simulink model "PMSM_FOC_Tractio"  (R2019b)
settings: Solver=FixedStepAuto  StartTime=0.0  StopTime=10  RelTol=1e-3
model workspace (MAT data in the model file):
  wc : Simulink.Parameter (value not decoded)
values from neighbouring files (symbols this model uses):
  CL_Param = tmp_CL_Param    [PMSM_Parameters.m]
  Cosine_table = [1,0.999995293095708,0.999990587122738,0.999985881149769,0.999981174245477,0.999967055395246,0.999952936545014,0.999938818626106,0.999924698844552,0.999901168979704,0.999877639114857,0.999854108318687,0.999830577522516,0.999797635711730,0.999764694832265,0.999731753021479,0.999698810279369,0.999656459316611,0.999614108353853,0.999571758322418,0.999529405497015,0.999477646313608,0.999425887130201,0 ...(+75635 chars)    [Motor_Table.m]
  ctrlParamsPI = tmp_ctrlParamsPI    [PMSM_Parameters.m]
  Flux_weak = tmp_Fluxweak_struct    [PMSM_Parameters.m]
  Hall_Parameter = tmp_Hall_struct    [PMSM_Parameters.m]
  HFI = tmp_HFI_struct    [PMSM_Parameters.m]
  inverter = struct    [PMSM_Parameters.m]
  MTPA_id_table = [-1.39452500000000,-1.36697494250000,-1.33970177000000,-1.31270548250000,-1.28598608000000,-1.25954356250000,-1.23337793000000,-1.20748918250000,-1.18187732000000,-1.15654234250000,-1.13148425000000,-1.10670304250000,-1.08219872000000,-1.05797128250000,-1.03402073000000,-1.01034706250000,-0.986950280000000,-0.963830382500000,-0.940987370000000,-0.918421242500000,-0.896132000000000,-0.8741196425000 ...(+3439 chars)    [Motor_Table.m]
  MTPA_iq_table = [-10.2740250000000,-10.1791705677750,-10.0840783722000,-9.98875081492500,-9.89319029760000,-9.79739922187500,-9.70137998940000,-9.60513500182500,-9.50866666080000,-9.41197736797500,-9.31506952500000,-9.21794553352500,-9.12060779520000,-9.02305871167500,-8.92530068460000,-8.82733611562500,-8.72916740640000,-8.63079695857500,-8.53222717380000,-8.43346045372500,-8.33449920000000,-8.23534581427500,-8. ...(+3121 chars)    [Motor_Table.m]
  MTPA_Te_Max = single(1.50)    [Motor_Table.m]
  MTPA_Te_Min = single(-1.50)    [Motor_Table.m]
  OPL_Param = tmp_OPL_Param    [PMSM_Parameters.m]
  pmsm = struct    [PMSM_Parameters.m]
  Resolver_Parameter = tmp_Resolver_struct    [PMSM_Parameters.m]
  Sine_table = [0,0.00153398793190718,0.00306797679513693,0.00460196565836668,0.00613595545291901,0.00766988657414913,0.00920381769537926,0.0107377488166094,0.0122716808691621,0.0138054965063930,0.0153393121436238,0.0168731296434999,0.0184069443494082,0.0199405867606401,0.0214742291718721,0.0230078706517816,0.0245415139943361,0.0260749254375696,0.0276083368808031,0.0291417483240366,0.0306751597672701,0.032208281 ...(+75648 chars)    [Motor_Table.m]
  SMO = temp_SMO    [PMSM_Parameters.m]
undefined symbols (not defined in the file or in its folder): DiscIntNeverNeededParam, Kiv, Kiw, Kpv, Kpw, magnitude, sigbuilder_block, SVPWM, Vdc
libraries: powerlib x29, fl_lib x18, simulink x10, nesl_utility x7, eeGeneralControl x4, dspstat3 x3, eeDiscretePi x2, powerlib_extras x1, ee_lib x1
(part 5 of 6)

== system PMSM_FOC_Tractio/Motor_Control/Motor_Control_Funtion/FOC_Control_100us/FOC/Angle_set/Subsystem/Subsystem1 ==
  HFI_Angle : Inport
  Action Port : ActionPort  ActionPortLabel=if(u1 ==3)
  Out1 : Outport
  wires:
  HFI_Angle/1 -> Out1/1

== system PMSM_FOC_Tractio/Motor_Control/Motor_Control_Funtion/FOC_Control_100us/FOC/Angle_set/Subsystem/Subsystem2 ==
  IPD_Angle : Inport
  Action Port : ActionPort  ActionPortLabel=elseif(u1 <3)
  Out1 : Outport
  wires:
  IPD_Angle/1 -> Out1/1

== system PMSM_FOC_Tractio/Motor_Control/Motor_Control_Funtion/FOC_Control_100us/FOC/Flux_weakening /Subsystem/Flux_weak ==
  note: sqrt(Ud*Ud+Uq*Uq)<=Udc/sqrt(3)
  Vd : Inport
  Vq : Inport  Port=2
  id_input : Inport  Port=3
  Iq_input : Inport  Port=4
  Add1 : Sum  OutDataTypeStr=Inherit: Same as first input
  Constant : Constant  Value=pmsm.RatedVoltage/sqrt(3)  OutDataTypeStr=single  SampleTime=-1
  Fcn : Fcn  Expr=sqrt(u(1)^2+u(2)^2)
  ID_Control : Subsystem
  Mux : Mux  Inputs=2
  Sum1 : Sum  Inputs=|-+
  Id_ref : Outport
  iq_ref : Outport  Port=2
  wires:
  Constant/1 -> Sum1/2
  Sum1/1 -> ID_Control/1(Err)
  Mux/1 -> Fcn/1
  Fcn/1 -> Sum1/1
  Vq/1 -> Mux/2
  Iq_input/1 -> iq_ref/1
  id_input/1 -> Add1/1
  Vd/1 -> Mux/1
  Add1/1 -> Id_ref/1
  ID_Control/1(PI_Out) -> Add1/2

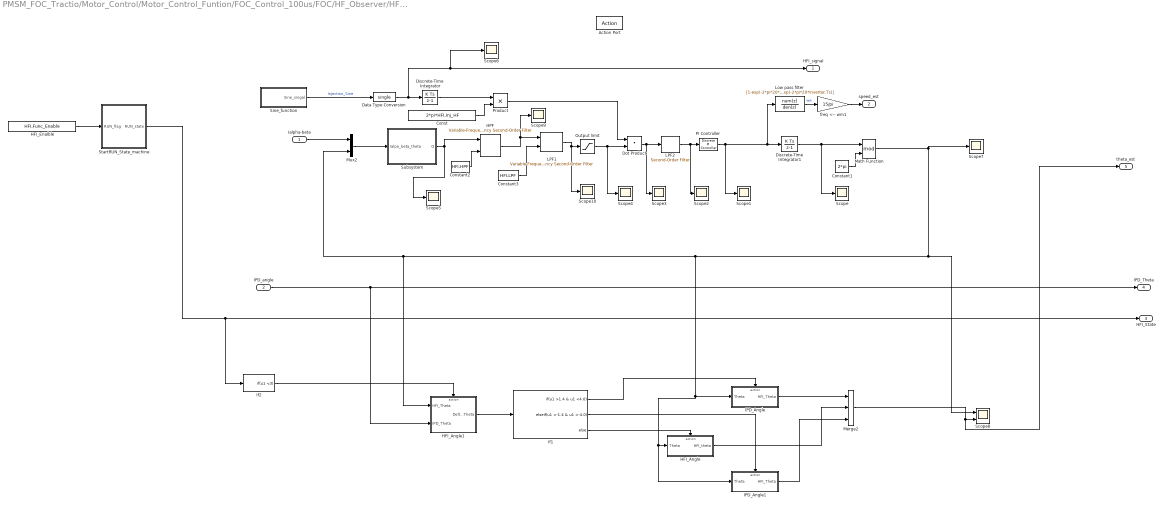
== system PMSM_FOC_Tractio/Motor_Control/Motor_Control_Funtion/FOC_Control_100us/FOC/HF_Observer/HFI_Function/HFI ==
  Ialpha-beta : Inport
  IPD_angle : Inport  Port=2
  Action Port : ActionPort  ActionPortLabel=case [ 3 ]:
  Const : Constant  Value=2*pi*HFI.Inj_HF  OutDataTypeStr=single
  Constant1 : Constant  Value=2*pi  OutDataTypeStr=single
  Constant2 : Constant  Value=HFI.HPF  OutDataTypeStr=single
  Constant3 : Constant  Value=HFI.LPF  OutDataTypeStr=single
  Data Type Conversion : DataTypeConversion  OutDataTypeStr=single
  Discrete-Time Integrator : DiscreteIntegrator  SampleTime=-1  ICPrevOutput=DiscIntNeverNeededParam  ICPrevScaledInput=DiscIntNeverNeededParam
  Discrete-Time Integrator1 : DiscreteIntegrator  SampleTime=-1  ICPrevOutput=DiscIntNeverNeededParam  ICPrevScaledInput=DiscIntNeverNeededParam
  Dot Product : DotProduct  InputSameDT=on  OutDataTypeStr=Inherit: Inherit via internal rule
  HFI_Angle : Subsystem
  HFI_Angle1 : Subsystem
  HFI_Enalble : Constant  Value=HFI.Func_Enable  OutDataTypeStr=uint8
  HPF : eeGeneralControl/Variable-Frequency Second-Order Filter  FilterType=High-pass  fn=HFI.HPF  Zeta=single(0.707)  Ts=-1  A0=0  Ph0=0  f0=0  b0=0
      settings: SourceProductName=Simscape Electrical  SourceProductBaseCode=PS
  IPD_Angle : Subsystem
  IPD_Angle1 : Subsystem
  If1 : If  IfExpression=u1 >1.4 & u1 <4.0  ElseIfExpressions=u1 <-1.4 & u1 >-4.0
  If2 : If  IfExpression=u1 <3  ShowElse=off
  LPF1 : eeGeneralControl/Variable-Frequency Second-Order Filter  FilterType=Low-pass  fn=HFI.LPF  Zeta=single(0.707)  Ts=-1  A0=0  Ph0=0  f0=0  b0=0
      settings: SourceProductName=Simscape Electrical  SourceProductBaseCode=PS
  LPF2 : eeGeneralControl/Second-Order Filter  FilterType=Low-pass  fn=100  Zeta=single(0.707)  Ts=-1  A0=0  Ph0=0  f0=0  b0=0
      settings: SourceProductName=Simscape Electrical  SourceProductBaseCode=PS
  Low pass filter : DiscreteTransferFcn  Numerator=[1-exp(-2*pi*20*inverter.Ts)]  Denominator=[1 -exp(-2*pi*20*inverter.Ts)]
  Math Function : Math  Operator=mod  SaturateOnIntegerOverflow=on
  Merge2 : Merge  Inputs=3
  Mux2 : Mux  Inputs=2
  Output limit : Saturate
  PI Controller : powerlib_extras/Discrete  Control Blocks/Discrete PI Controller  Kp=HFI.PI_Kp  Ki=HFI.PI_Ki  Par_Limits=[100*2*pi -100*2*pi]  Init=0  Ts=-1
      settings: SourceProductName=Simscape Electrical
  Product : Product
  Scope{,1..7,9..10} (10 alike) : Scope
  Scope8 : Scope  NumInputPorts=2
  Sine_function : Subsystem
      settings: RTWSystemCode=Nonreusable function  RTWFcnNameOpts=Use subsystem name
  StartRUN_State_machine : Stateflow chart  BlockKeywords=__PRM__SERIALIZED__DATA__:Stateflow Chart,Stateflow Diagram  TreatAsAtomicUnit=on
      settings: RTWSystemCode=Nonreusable function  RTWFcnNameOpts=Use subsystem name
  Subsystem : Subsystem
  freq <-- wm1 : Gain  Gain=15/pi
  HFI_signal : Outport
  speed_est : Outport  Port=2
  HFI_State : Outport  Port=3
  IPD_Theta : Outport  Port=4
  theta_est : Outport  Port=5
  wires:
  Mux2/1 -> Subsystem/1(Ialpa_beta_theta)
  Ialpha-beta/1 -> Mux2/1
  Subsystem/1(Q) -> HPF/1, Scope5/1
  freq <-- wm1/1 -> speed_est/1
  Discrete-Time Integrator1/1 -> Scope/1, Math Function/1
  LPF1/1 -> Scope10/1, Output limit/1
  LPF2/1 -> Scope2/1, PI Controller/1
  Low pass filter/1 -> freq <-- wm1/1  "we"
  HPF/1 -> LPF1/1, Scope9/1
  Discrete-Time Integrator/1 -> Product/1
  Product/1 -> Dot Product/1
  Dot Product/1 -> LPF2/1, Scope3/1
  Constant1/1 -> Math Function/2
  Output limit/1 -> Scope4/1, Dot Product/2
  Const/1 -> Product/2
  Sine_function/1(Sine_singal) -> Data Type Conversion/1  "Injection_Sine"
  Data Type Conversion/1 -> Scope6/1, HFI_signal/1, Discrete-Time Integrator/1
  HFI_Enalble/1 -> StartRUN_State_machine/1(RUN_flag)
  StartRUN_State_machine/1(RUN_state) -> If2/1, HFI_State/1
  IPD_angle/1 -> HFI_Angle1/2(IPD_Theta), IPD_Theta/1
  Math Function/1 -> IPD_Angle1/1(Theta), HFI_Angle/1(Theta), IPD_Angle/1(Theta), HFI_Angle1/1(HFI_Theta), Mux2/2, Scope8/1, Scope7/1
  PI Controller/1 -> Low pass filter/1, Discrete-Time Integrator1/1, Scope1/1
  If1/1 -> IPD_Angle/Action
  HFI_Angle/1(HFI_theta) -> Merge2/2
  If1/3 -> HFI_Angle/Action
  IPD_Angle/1(HFI_Theta) -> Merge2/1
  HFI_Angle1/1(Delta_Theta) -> If1/1
  If2/1 -> HFI_Angle1/Action
  Merge2/1 -> theta_est/1, Scope8/2
  If1/2 -> IPD_Angle1/Action
  IPD_Angle1/1(HFI_Theta) -> Merge2/3
  Constant2/1 -> HPF/2
  Constant3/1 -> LPF1/2

== system PMSM_FOC_Tractio/Motor_Control/Motor_Control_Funtion/FOC_Control_100us/FOC/HF_Observer/HFI_Function/IPD ==
  Iabc : Inport  PortDimensions=3
  Action Port : ActionPort  ActionPortLabel=case [ 1 ]:
  7 : Fcn  Expr=u[1]*u[3]
  8 : Fcn  Expr=u[1]*u[2]
  Constant : Constant  Value=HFI.IPD_V
  Demux1 : Demux  Outputs=3
  HF_Angle : Subsystem
  Mux : Mux  Inputs=3
  Scope : Scope
  Sine_Cosine : Subsystem  TreatAsAtomicUnit=on
      settings: RTWSystemCode=Nonreusable function  RTWFcnNameOpts=Use subsystem name
  Theta_cacl : Subsystem
      settings: RTWSystemCode=Nonreusable function
  Ualpha : Outport
  Ubeta : Outport  Port=2
  Theta : Outport  Port=3
  wires:
  Sine_Cosine/1(Sin) -> Mux/2
  Sine_Cosine/2(Cos) -> Mux/3
  Constant/1 -> Mux/1
  Mux/1 -> 8/1, 7/1
  7/1 -> Ualpha/1
  8/1 -> Ubeta/1
  Iabc/1 -> Scope/1, Demux1/1  "Phase_CurrentABC"
  HF_Angle/1(Theta_V) -> Sine_Cosine/1(P)
  Demux1/3 -> Theta_cacl/3(Ic)
  Demux1/2 -> Theta_cacl/2(Ib)
  Theta_cacl/1(Theta) -> Theta/1
  Demux1/1 -> Theta_cacl/1(Ia)

== system PMSM_FOC_Tractio/Motor_Control/Motor_Control_Funtion/FOC_Control_100us/FOC/HF_Observer/HFI_Function/NS ==
  Id : Inport
  Theta : Inport  Port=2
  Action Port : ActionPort  ActionPortLabel=case [ 2 ]:
  Abs : Abs
  Abs1 : Abs
  Data Type Conversion : DataTypeConversion
  Delay : Delay  DelayLength=1  InitialCondition=0
  Delay1 : Delay  DelayLength=1  InitialCondition=0
  HFI_Enalble : Constant  Value=HFI.Func_Enable  OutDataTypeStr=uint8
  Merge : Merge  Inputs=5
  Merge1 : Merge  Inputs=5
  NS_State_machine : Stateflow chart  BlockKeywords=__PRM__SERIALIZED__DATA__:Stateflow Chart,Stateflow Diagram  TreatAsAtomicUnit=on
      settings: RTWSystemCode=Nonreusable function  RTWFcnNameOpts=Use subsystem name
  Scope1 : Scope  NumInputPorts=2
  Switch Case1 : SwitchCase  CaseConditions={1,2,3,4,5}  ShowDefaultCase=off
  Ud_inject_1 : Subsystem
  Ud_inject_2 : Subsystem
  Ud_inject_3 : Subsystem
  Ud_inject_4 : Subsystem
  Ud_inject_5 : Subsystem
  Ualpha : Outport
  Ubeta : Outport  Port=2
  IPD_Angle : Outport  Port=3
  Angle_RUN : Outport  Port=4
  wires:
  HFI_Enalble/1 -> NS_State_machine/1(NS_flag1)
  NS_State_machine/1(NS_state) -> Switch Case1/1
  Id/1 -> Ud_inject_2/1(Id), Ud_inject_4/1(Id)
  Merge/1 -> Scope1/1, Ualpha/1
  Ud_inject_2/1(Ualpha) -> Merge/1
  Ud_inject_4/1(Ualpha) -> Merge/2
  Merge1/1 -> Scope1/2, Ubeta/1
  Ud_inject_2/2(Ubeta) -> Merge1/1
  Ud_inject_4/2(Ubeta) -> Merge1/2
  Ud_inject_4/3(Id_out) -> Delay1/1
  Ud_inject_2/3(Id_out) -> Delay/1
  Ud_inject_1/1(Ualpha) -> Merge/3
  Ud_inject_1/2(Ubeta) -> Merge1/3
  Ud_inject_3/1(Ualpha) -> Merge/4
  Ud_inject_3/2(Ubeta) -> Merge1/4
  Switch Case1/1 -> Ud_inject_1/Action
  Switch Case1/2 -> Ud_inject_2/Action
  Theta/1 -> Ud_inject_4/2(Theta), Ud_inject_2/2(Theta), Ud_inject_1/1(Theta), Ud_inject_5/1(Theta), Ud_inject_3/1(Theta)
  Switch Case1/3 -> Ud_inject_3/Action
  Switch Case1/4 -> Ud_inject_4/Action
  Switch Case1/5 -> Ud_inject_5/Action
  Ud_inject_5/1(Ualpha) -> Merge/5
  Ud_inject_5/2(Ubeta) -> Merge1/5
  Abs/1 -> Ud_inject_5/2(Id1)
  Abs1/1 -> Ud_inject_5/3(Id2)
  Ud_inject_5/3(IPD_Angle) -> Data Type Conversion/1, IPD_Angle/1
  Delay/1 -> Abs/1
  Delay1/1 -> Abs1/1
  Data Type Conversion/1 -> Angle_RUN/1

== system PMSM_FOC_Tractio/Motor_Control/Motor_Control_Funtion/Angle_Speed_100us/SpeedAndAngle/ACC_OMG/BLDC/Control/Commutation ==
  Hall : Inport
  Bias : Bias  Bias=-1
  Bit concatenate : Subsystem
  Data Type Conversion : DataTypeConversion
  Direct Lookup Table (n-D)2 : LookupNDDirect  InputsSelectThisObjectFromTable=Vector  Table=[0 0 0 1 1 0;0 1 1 0 0 0;0 1 0 0 0 1;1 0 0 0 1 0;1 0 1 0 0 0;0 0 0 1 0 1]
  Scope : Scope
  S : Outport  VectorParamsAs1DForOutWhenUnconnected=off
  wires:
  Hall/1 -> Bit concatenate/1(u)
  Bit concatenate/1(y) -> Data Type Conversion/1
  Direct Lookup Table (n-D)2/1 -> S/1
  Data Type Conversion/1 -> Bias/1
  Bias/1 -> Scope/1, Direct Lookup Table (n-D)2/1

== system PMSM_FOC_Tractio/Motor_Control/Motor_Control_Funtion/Angle_Speed_100us/SpeedAndAngle/ACC_OMG/BLDC/Control/Speed_Control ==
  Err : Inport
  Action Port : ActionPort  ActionPortLabel=if(u1==3)
  Add : Sum
  Cons : Constant  Value=0  OutDataTypeStr=single
  Discrete-Time Integrator : DiscreteIntegrator  SampleTime=-1  ICPrevOutput=DiscIntNeverNeededParam  ICPrevScaledInput=DiscIntNeverNeededParam
  Ki : Constant  Value=17.72  OutDataTypeStr=single
  Kp : Constant  Value=0.7476  OutDataTypeStr=single
  Product : Product
  Product1 : Product
  Relational Operator1 : RelationalOperator  Operator===  OutDataTypeStr=boolean  RndMeth=Simplest
  Saturation : Saturate  UpperLimit=4200  LowerLimit=0
  Scope : Scope
  Switch : Switch  Criteria=u2 > Threshold
  Unit Delay3 : UnitDelay  SampleTime=-1  HasFrameUpgradeWarning=on
  PI_Out : Outport
  wires:
  Kp/1 -> Product/1
  Err/1 -> Switch/1, Product/2
  Switch/1 -> Product1/2
  Product1/1 -> Discrete-Time Integrator/1
  Product/1 -> Add/1
  Add/1 -> Relational Operator1/1, Saturation/1
  Saturation/1 -> Relational Operator1/2, PI_Out/1
  Discrete-Time Integrator/1 -> Add/2, Scope/1
  Relational Operator1/1 -> Unit Delay3/1
  Ki/1 -> Product1/1
  Unit Delay3/1 -> Switch/2
  Cons/1 -> Switch/3

== system PMSM_FOC_Tractio/Motor_Control/Motor_Control_Funtion/Angle_Speed_100us/SpeedAndAngle/Subsystem/Subsystem1/Commutation/Bit concatenate ==
  u : Inport
  Gain : Gain  Gain=[4 2 1]  Multiplication=Matrix(K*u)
  Sum of Elements : Sum  Inputs=+
  y : Outport  VectorParamsAs1DForOutWhenUnconnected=off
  wires:
  u/1 -> Gain/1
  Gain/1 -> Sum of Elements/1
  Sum of Elements/1 -> y/1

== system PMSM_FOC_Tractio/Motor_Control/Motor_Control_Funtion/FOC_Control_100us/FOC/Flux_weakening /Subsystem/Flux_weak/ID_Control ==
  Err : Inport
  Add : Sum
  Cons : Constant  Value=0  OutDataTypeStr=single
  Discrete-Time Integrator : DiscreteIntegrator  SampleTime=-1  ICPrevOutput=DiscIntNeverNeededParam  ICPrevScaledInput=DiscIntNeverNeededParam
  Ki : Constant  Value=ki  OutDataTypeStr=single
  Kp : Constant  Value=kp  OutDataTypeStr=single
  Product : Product
  Product1 : Product
  Relational Operator1 : RelationalOperator  Operator===  OutDataTypeStr=boolean  RndMeth=Simplest
  Saturation : Saturate  UpperLimit=Id_max  LowerLimit=Id_min
  Switch : Switch  Criteria=u2 > Threshold
  Unit Delay3 : UnitDelay  SampleTime=-1  HasFrameUpgradeWarning=on
  PI_Out : Outport
  wires:
  Kp/1 -> Product/1
  Err/1 -> Switch/1, Product/2
  Switch/1 -> Product1/2
  Product1/1 -> Discrete-Time Integrator/1
  Product/1 -> Add/1
  Add/1 -> Relational Operator1/1, Saturation/1
  Saturation/1 -> Relational Operator1/2, PI_Out/1
  Cons/1 -> Switch/3
  Discrete-Time Integrator/1 -> Add/2
  Relational Operator1/1 -> Unit Delay3/1
  Ki/1 -> Product1/1
  Unit Delay3/1 -> Switch/2

== system PMSM_FOC_Tractio/Motor_Control/Motor_Control_Funtion/FOC_Control_100us/FOC/HF_Observer/HFI_Function/HFI/HFI_Angle ==
  Theta : Inport
  Action Port : ActionPort  ActionPortLabel=else
  HFI_theta : Outport
  wires:
  Theta/1 -> HFI_theta/1

== system PMSM_FOC_Tractio/Motor_Control/Motor_Control_Funtion/FOC_Control_100us/FOC/HF_Observer/HFI_Function/HFI/HFI_Angle1 ==
  HFI_Theta : Inport
  IPD_Theta : Inport  Port=2
  Action Port : ActionPort  ActionPortLabel=if(u1 <3)
  Subtract : Sum  Inputs=+-
  Delta_Theta : Outport
  wires:
  HFI_Theta/1 -> Subtract/1
  IPD_Theta/1 -> Subtract/2
  Subtract/1 -> Delta_Theta/1

== system PMSM_FOC_Tractio/Motor_Control/Motor_Control_Funtion/FOC_Control_100us/FOC/HF_Observer/HFI_Function/HFI/IPD_Angle ==
  Theta : Inport
  Action Port : ActionPort  ActionPortLabel=if(u1 >1.4 & u1 <4.0)
  Angle_calibration : Subsystem  TreatAsAtomicUnit=on
      settings: RTWSystemCode=Nonreusable function  RTWFcnNameOpts=Use subsystem name
  HFI_Theta : Outport
  wires:
  Theta/1 -> Angle_calibration/1(Angle_input)
  Angle_calibration/1(Angle_output) -> HFI_Theta/1

== system PMSM_FOC_Tractio/Motor_Control/Motor_Control_Funtion/FOC_Control_100us/FOC/HF_Observer/HFI_Function/HFI/IPD_Angle1 ==
  Theta : Inport
  Action Port : ActionPort  ActionPortLabel=elseif(u1 <-1.4 & u1 >-4.0)
  Angle_calibration : Subsystem  TreatAsAtomicUnit=on
      settings: RTWSystemCode=Nonreusable function  RTWFcnNameOpts=Use subsystem name
  HFI_Theta : Outport
  wires:
  Theta/1 -> Angle_calibration/1(Angle_input)
  Angle_calibration/1(Angle_output) -> HFI_Theta/1

== system PMSM_FOC_Tractio/Motor_Control/Motor_Control_Funtion/FOC_Control_100us/FOC/HF_Observer/HFI_Function/HFI/Sine_function ==
  A : Gain  Gain=HFI.Inj_HV
  Add : Sum
  Const1 : Constant  Value=2*pi*inverter.Ts*HFI.Inj_HF  OutDataTypeStr=single
  Const2 : Constant  Value=2*pi  OutDataTypeStr=single
  Const3 : Constant  Value=0  OutDataTypeStr=single
  Const4 : Constant  OutDataTypeStr=single
  Delay : Delay  DelayLength=1  InitialCondition=0
  Memory : Memory  InheritSampleTime=on
  Product1 : Product
  Relational Operator1 : RelationalOperator  Operator=<  OutDataTypeStr=boolean  RndMeth=Simplest
  Sine : Lookup_n-D  NumberOfTableDimensions=1  LookupTableObject=''  BreakpointsForDimension1=[0:2*pi/4095:2*pi]  BreakpointsForDimension1FirstPoint=10  BreakpointsForDimension2FirstPoint=10  BreakpointsForDimension1Spacing=12  BreakpointsForDimension2Spacing=12  IndexSearchMethod=Evenly spaced points  Table=Sine_table  InterpMethod=Flat  DiagnosticForOutOfRangeInput=Error  InternalRulePriority=Speed  RndMeth=Simplest  InputSameDT=on
  Switch : Switch  Criteria=u2 > Threshold
  Sine_singal : Outport
  wires:
  Switch/1 -> Product1/1
  Const3/1 -> Switch/3
  Relational Operator1/1 -> Switch/2
  Delay/1 -> Relational Operator1/1
  Const2/1 -> Relational Operator1/2
  Add/1 -> Memory/1, Delay/1
  Sine/1 -> A/1
  Product1/1 -> Sine/1, Add/2
  Memory/1 -> Product1/2
  Const1/1 -> Add/1
  Const4/1 -> Switch/1
  A/1 -> Sine_singal/1

== system PMSM_FOC_Tractio/Motor_Control/Motor_Control_Funtion/FOC_Control_100us/FOC/HF_Observer/HFI_Function/HFI/Subsystem ==
  Ialpa_beta_theta : Inport
  Add2 : Sum  Inputs=-+  OutDataTypeStr=Inherit: Same as first input
  Demux : Demux  Outputs=2
  Demux1 : Demux  Outputs=2
  Produc3t : Product  RndMeth=Simplest  OutDataTypeStr=Inherit: Same as first input
  Product4 : Product  RndMeth=Simplest  OutDataTypeStr=Inherit: Same as first input
  Sine_Cosine : Subsystem
      settings: RTWSystemCode=Nonreusable function  RTWFcnNameOpts=Use subsystem name
  Q : Outport  VectorParamsAs1DForOutWhenUnconnected=off
  wires:
  Add2/1 -> Q/1
  Sine_Cosine/2(Cos) -> Product4/2
  Produc3t/1 -> Add2/1
  Sine_Cosine/1(Sin) -> Produc3t/2
  Product4/1 -> Add2/2
  Demux/1 -> Produc3t/1
  Demux/2 -> Product4/1
  Demux1/1 -> Demux/1
  Demux1/2 -> Sine_Cosine/1(P)
  Ialpa_beta_theta/1 -> Demux1/1

== system PMSM_FOC_Tractio/Motor_Control/Motor_Control_Funtion/FOC_Control_100us/FOC/HF_Observer/HFI_Function/IPD/HF_Angle ==
  Add : Sum
  Const1 : Constant  Value=2*pi*inverter.Ts*HFI.IPD_F  OutDataTypeStr=single
  Const2 : Constant  Value=2*pi  OutDataTypeStr=single
  Const3 : Constant  Value=0  OutDataTypeStr=single
  Const4 : Constant  OutDataTypeStr=single
  Delay : Delay  DelayLength=1  InitialCondition=0
  Memory : Memory  InheritSampleTime=on
  Product1 : Product
  Relational Operator1 : RelationalOperator  Operator=<  OutDataTypeStr=boolean  RndMeth=Simplest
  Switch : Switch  Criteria=u2 > Threshold
  Theta_V : Outport
  wires:
  Switch/1 -> Product1/1
  Delay/1 -> Relational Operator1/1
  Const2/1 -> Relational Operator1/2
  Const3/1 -> Switch/3
  Relational Operator1/1 -> Switch/2
  Const1/1 -> Add/1
  Memory/1 -> Product1/2
  Add/1 -> Memory/1, Delay/1
  Product1/1 -> Theta_V/1, Add/2
  Const4/1 -> Switch/1

== system PMSM_FOC_Tractio/Motor_Control/Motor_Control_Funtion/FOC_Control_100us/FOC/HF_Observer/HFI_Function/IPD/Sine_Cosine ==
  note: Sine Cosine Coefficients
  P : Inport
  Cosine : Lookup_n-D  NumberOfTableDimensions=1  LookupTableObject=''  BreakpointsForDimension1=[0:2*pi/4095:2*pi]  BreakpointsForDimension1FirstPoint=10  BreakpointsForDimension2FirstPoint=10  BreakpointsForDimension1Spacing=12  BreakpointsForDimension2Spacing=12  IndexSearchMethod=Evenly spaced points  Table=Cosine_table  InterpMethod=Flat  DiagnosticForOutOfRangeInput=Error  InternalRulePriority=Speed  RndMeth=Simplest  InputSameDT=on
  Scope : Scope  NumInputPorts=2
  Sine : Lookup_n-D  NumberOfTableDimensions=1  LookupTableObject=''  BreakpointsForDimension1=[0:2*pi/4095:2*pi]  BreakpointsForDimension1FirstPoint=10  BreakpointsForDimension2FirstPoint=10  BreakpointsForDimension1Spacing=12  BreakpointsForDimension2Spacing=12  IndexSearchMethod=Evenly spaced points  Table=Sine_table  InterpMethod=Flat  DiagnosticForOutOfRangeInput=Error  InternalRulePriority=Speed  RndMeth=Simplest  InputSameDT=on
  Sin : Outport  VectorParamsAs1DForOutWhenUnconnected=off
  Cos : Outport  Port=2  VectorParamsAs1DForOutWhenUnconnected=off
  wires:
  P/1 -> Cosine/1, Sine/1  "position"
  Sine/1 -> Scope/1, Sin/1
  Cosine/1 -> Scope/2, Cos/1

== system PMSM_FOC_Tractio/Motor_Control/Motor_Control_Funtion/FOC_Control_100us/FOC/HF_Observer/HFI_Function/IPD/Theta_cacl ==
  Ia : Inport
  Ib : Inport  Port=2
  Ic : Inport  Port=3
  Display{1..3,6} (4 alike) : Display
  Gain1 : Gain  Gain=pi/180
  If Action Subsystem1 : Subsystem  TreatAsAtomicUnit=on
  If Action Subsystem2 : Subsystem  TreatAsAtomicUnit=on
  If Action Subsystem3 : Subsystem  TreatAsAtomicUnit=on
  If Action Subsystem4 : Subsystem  TreatAsAtomicUnit=on
  If Action Subsystem5 : Subsystem  TreatAsAtomicUnit=on
  If Action Subsystem6 : Subsystem  TreatAsAtomicUnit=on
  If1 : If  NumInputs=3  IfExpression=(u1>u3)&(u3>u2)  ElseIfExpressions=(u3>u1)&(u1>u2),(u3>u2)&(u2>u1),(u2>u3)&(u3>u1),(u2>u1)&(u1>u3),(u1>u2)&(u2>u3)  ShowElse=off
  Merge : Merge  Inputs=6
  Mux2 : Mux  Inputs=3
  RMS : dspstat3/RMS  run=on  directionMode=Each column  dimension=1  reset_popup=None
  RMS1 : dspstat3/RMS  run=on  directionMode=Each column  dimension=1  reset_popup=None
  RMS2 : dspstat3/RMS  run=on  directionMode=Each column  dimension=1  InputProcessing=Columns as channels (frame based)  reset_popup=None
  Scope1 : Scope  NumInputPorts=3
  Scope2 : Scope  NumInputPorts=3
  Theta : Outport
  wires:
  Ia/1 -> Scope2/1, RMS/1
  Ib/1 -> Scope2/2, RMS1/1
  Ic/1 -> Scope2/3, RMS2/1
  RMS2/1 -> Mux2/3, If1/3, Display3/1, Scope1/3
  RMS1/1 -> Mux2/2, If1/2, Display2/1, Scope1/2
  RMS/1 -> If1/1, Mux2/1, Display1/1, Scope1/1
  If1/1 -> If Action Subsystem2/Action
  If1/2 -> If Action Subsystem1/Action
  If1/3 -> If Action Subsystem3/Action
  If1/4 -> If Action Subsystem4/Action
  If1/5 -> If Action Subsystem5/Action
  If1/6 -> If Action Subsystem6/Action
  Mux2/1 -> If Action Subsystem6/1(In1), If Action Subsystem5/1(In1), If Action Subsystem4/1(In1), If Action Subsystem3/1(In1), If Action Subsystem1/1(In1), If Action Subsystem2/1(In1)
  If Action Subsystem2/1(Out1) -> Merge/1
  If Action Subsystem1/1(Out1) -> Merge/2
  If Action Subsystem3/1(Out1) -> Merge/3
  If Action Subsystem4/1(Out1) -> Merge/4
  If Action Subsystem5/1(Out1) -> Merge/5
  If Action Subsystem6/1(Out1) -> Merge/6
  Merge/1 -> Gain1/1
  Gain1/1 -> Display6/1, Theta/1

== system PMSM_FOC_Tractio/Motor_Control/Motor_Control_Funtion/FOC_Control_100us/FOC/HF_Observer/HFI_Function/NS/Ud_inject_1 ==
  Theta : Inport
  Action Port : ActionPort  ActionPortLabel=case [ 1 ]:
  1 : Fcn  Expr=u[1]*u[4]-u[2]*u[3]
  2 : Fcn  Expr=u[1]*u[3]+u[2]*u[4]
  Constant : Constant  Value=0  OutDataTypeStr=single
  Constant2 : Constant  Value=0  OutDataTypeStr=single
  Mux : Mux
  Sine_Cosine : Subsystem  TreatAsAtomicUnit=on
      settings: RTWSystemCode=Nonreusable function  RTWFcnNameOpts=Use subsystem name
  Ualpha : Outport
  Ubeta : Outport  Port=2
  wires:
  Constant2/1 -> Mux/2
  Theta/1 -> Sine_Cosine/1(P)
  2/1 -> Ubeta/1
  Sine_Cosine/2(Cos) -> Mux/4
  1/1 -> Ualpha/1
  Constant/1 -> Mux/1
  Mux/1 -> 2/1, 1/1
  Sine_Cosine/1(Sin) -> Mux/3

== system PMSM_FOC_Tractio/Motor_Control/Motor_Control_Funtion/FOC_Control_100us/FOC/HF_Observer/HFI_Function/NS/Ud_inject_2 ==
  Id : Inport
  Theta : Inport  Port=2
  Action Port : ActionPort  ActionPortLabel=case [ 2 ]:
  1 : Fcn  Expr=u[1]*u[4]-u[2]*u[3]
  2 : Fcn  Expr=u[1]*u[3]+u[2]*u[4]
  Constant : Constant  Value=HFI.NS_V  OutDataTypeStr=single
  Constant2 : Constant  Value=0  OutDataTypeStr=single
  Mux : Mux
  Sine_Cosine : Subsystem  TreatAsAtomicUnit=on
      settings: RTWSystemCode=Nonreusable function  RTWFcnNameOpts=Use subsystem name
  Ualpha : Outport
  Ubeta : Outport  Port=2
  Id_out : Outport  Port=3
  wires:
  Constant2/1 -> Mux/2
  Theta/1 -> Sine_Cosine/1(P)
  2/1 -> Ubeta/1
  Sine_Cosine/2(Cos) -> Mux/4
  1/1 -> Ualpha/1
  Constant/1 -> Mux/1
  Mux/1 -> 2/1, 1/1
  Sine_Cosine/1(Sin) -> Mux/3
  Id/1 -> Id_out/1

== system PMSM_FOC_Tractio/Motor_Control/Motor_Control_Funtion/FOC_Control_100us/FOC/HF_Observer/HFI_Function/NS/Ud_inject_3 ==
  Theta : Inport
  Action Port : ActionPort  ActionPortLabel=case [ 3 ]:
  1 : Fcn  Expr=u[1]*u[4]-u[2]*u[3]
  2 : Fcn  Expr=u[1]*u[3]+u[2]*u[4]
  Constant : Constant  Value=0  OutDataTypeStr=single
  Constant2 : Constant  Value=0  OutDataTypeStr=single
  Mux : Mux
  Sine_Cosine : Subsystem  TreatAsAtomicUnit=on
      settings: RTWSystemCode=Nonreusable function  RTWFcnNameOpts=Use subsystem name
  Ualpha : Outport
  Ubeta : Outport  Port=2
  wires:
  Constant2/1 -> Mux/2
  Theta/1 -> Sine_Cosine/1(P)
  2/1 -> Ubeta/1
  Sine_Cosine/2(Cos) -> Mux/4
  1/1 -> Ualpha/1
  Constant/1 -> Mux/1
  Mux/1 -> 2/1, 1/1
  Sine_Cosine/1(Sin) -> Mux/3

== system PMSM_FOC_Tractio/Motor_Control/Motor_Control_Funtion/FOC_Control_100us/FOC/HF_Observer/HFI_Function/NS/Ud_inject_4 ==
  Id : Inport
  Theta : Inport  Port=2
  Action Port : ActionPort  ActionPortLabel=case [ 4 ]:
  1 : Fcn  Expr=u[1]*u[4]-u[2]*u[3]
  2 : Fcn  Expr=u[1]*u[3]+u[2]*u[4]
  Constant : Constant  Value=HFI.NS_V  OutDataTypeStr=single
  Constant2 : Constant  Value=0  OutDataTypeStr=single
  Mux : Mux
  Sine_Cosine : Subsystem  TreatAsAtomicUnit=on
      settings: RTWSystemCode=Nonreusable function
  Theta_limit : Subsystem
      settings: RTWSystemCode=Nonreusable function
  Ualpha : Outport
  Ubeta : Outport  Port=2
  Id_out : Outport  Port=3
  wires:
  Constant2/1 -> Mux/2
  2/1 -> Ubeta/1
  Sine_Cosine/2(Cos) -> Mux/4
  1/1 -> Ualpha/1
  Constant/1 -> Mux/1
  Mux/1 -> 2/1, 1/1
  Sine_Cosine/1(Sin) -> Mux/3
  Id/1 -> Id_out/1
  Theta_limit/1(Angle_output) -> Sine_Cosine/1(P)
  Theta/1 -> Theta_limit/1(Angle_input)

== system PMSM_FOC_Tractio/Motor_Control/Motor_Control_Funtion/FOC_Control_100us/FOC/HF_Observer/HFI_Function/NS/Ud_inject_5 ==
  Theta : Inport
  Id1 : Inport  Port=2
  Id2 : Inport  Port=3
  Action Port : ActionPort  ActionPortLabel=case [ 5 ]:
  1 : Fcn  Expr=u[1]*u[4]-u[2]*u[3]
  2 : Fcn  Expr=u[1]*u[3]+u[2]*u[4]
  Constant : Constant  Value=0  OutDataTypeStr=single
  Constant2 : Constant  Value=0  OutDataTypeStr=single
  If1 : If  NumInputs=2  IfExpression=u1>=u2  ElseIfExpressions=u1<u2  ShowElse=off
  Merge1 : Merge
  Mux : Mux
  Sine_Cosine : Subsystem
      settings: RTWSystemCode=Nonreusable function  RTWFcnNameOpts=Use subsystem name
  Subsystem : Subsystem
  Subsystem1 : Subsystem
  Ualpha : Outport
  Ubeta : Outport  Port=2
  IPD_Angle : Outport  Port=3
  wires:
  Constant2/1 -> Mux/2
  Theta/1 -> Subsystem1/1(In1), Subsystem/1(In1), Sine_Cosine/1(P)
  2/1 -> Ubeta/1
  Sine_Cosine/2(Cos) -> Mux/4
  1/1 -> Ualpha/1
  Constant/1 -> Mux/1
  Mux/1 -> 2/1, 1/1
  Sine_Cosine/1(Sin) -> Mux/3
  Id1/1 -> If1/1
  Id2/1 -> If1/2
  If1/1 -> Subsystem/Action
  If1/2 -> Subsystem1/Action
  Subsystem/1(Out1) -> Merge1/1
  Subsystem1/1(Out1) -> Merge1/2
  Merge1/1 -> IPD_Angle/1

== system PMSM_FOC_Tractio/Motor_Control/Motor_Control_Funtion/Angle_Speed_100us/SpeedAndAngle/ACC_OMG/BLDC/Control/Commutation/Bit concatenate ==
  u : Inport
  Gain : Gain  Gain=[4 2 1]  Multiplication=Matrix(K*u)
  Sum of Elements : Sum  Inputs=+
  y : Outport  VectorParamsAs1DForOutWhenUnconnected=off
  wires:
  u/1 -> Gain/1
  Gain/1 -> Sum of Elements/1
  Sum of Elements/1 -> y/1

== system PMSM_FOC_Tractio/Motor_Control/Motor_Control_Funtion/FOC_Control_100us/FOC/HF_Observer/HFI_Function/HFI/IPD_Angle/Angle_calibration ==
  Angle_input : Inport
  Angle_offset : Constant  Value=-pi  OutDataTypeStr=single
  If Action Subsystem1 : Subsystem  TreatAsAtomicUnit=on
  If Action Subsystem2 : Subsystem  TreatAsAtomicUnit=on
  If Action Subsystem3 : Subsystem  TreatAsAtomicUnit=on
  If1 : If  IfExpression=u1 > 6.283185307  ElseIfExpressions=u1<0
  Merge1 : Merge  Inputs=3
  Subtract1 : Sum
  Angle_output : Outport
  wires:
  Angle_input/1 -> Subtract1/1
  Angle_offset/1 -> Subtract1/2  "Control_ModeCommand"
  If1/1 -> If Action Subsystem2/Action
  If1/3 -> If Action Subsystem1/Action
  If Action Subsystem2/1(Out1) -> Merge1/1
  Subtract1/1 -> If Action Subsystem3/1(In1), If Action Subsystem1/1(In1), If Action Subsystem2/1(In1), If1/1
  If Action Subsystem1/1(Out1) -> Merge1/3
  If Action Subsystem3/1(Out1) -> Merge1/2
  If1/2 -> If Action Subsystem3/Action
  Merge1/1 -> Angle_output/1

== system PMSM_FOC_Tractio/Motor_Control/Motor_Control_Funtion/FOC_Control_100us/FOC/HF_Observer/HFI_Function/HFI/IPD_Angle1/Angle_calibration ==
  Angle_input : Inport
  Angle_offset : Constant  Value=pi  OutDataTypeStr=single
  If Action Subsystem1 : Subsystem  TreatAsAtomicUnit=on
  If Action Subsystem2 : Subsystem  TreatAsAtomicUnit=on
  If Action Subsystem3 : Subsystem  TreatAsAtomicUnit=on
  If1 : If  IfExpression=u1 > 6.283185307  ElseIfExpressions=u1<0
  Merge1 : Merge  Inputs=3
  Subtract1 : Sum
  Angle_output : Outport
  wires:
  Angle_input/1 -> Subtract1/1
  Angle_offset/1 -> Subtract1/2  "Control_ModeCommand"
  If1/1 -> If Action Subsystem2/Action
  If1/3 -> If Action Subsystem1/Action
  If Action Subsystem2/1(Out1) -> Merge1/1
  Subtract1/1 -> If Action Subsystem3/1(In1), If Action Subsystem1/1(In1), If Action Subsystem2/1(In1), If1/1
  If Action Subsystem1/1(Out1) -> Merge1/3
  If Action Subsystem3/1(Out1) -> Merge1/2
  If1/2 -> If Action Subsystem3/Action
  Merge1/1 -> Angle_output/1

== system PMSM_FOC_Tractio/Motor_Control/Motor_Control_Funtion/FOC_Control_100us/FOC/HF_Observer/HFI_Function/HFI/Subsystem/Sine_Cosine ==
  note: Sine Cosine Coefficients
  P : Inport
  Cosine : Lookup_n-D  NumberOfTableDimensions=1  LookupTableObject=''  BreakpointsForDimension1=[0:2*pi/4095:2*pi]  BreakpointsForDimension1FirstPoint=10  BreakpointsForDimension2FirstPoint=10  BreakpointsForDimension1Spacing=12  BreakpointsForDimension2Spacing=12  IndexSearchMethod=Evenly spaced points  Table=Cosine_table  InterpMethod=Flat  DiagnosticForOutOfRangeInput=Error  InternalRulePriority=Speed  RndMeth=Simplest  InputSameDT=on
  Saturation : Saturate  UpperLimit=2*pi-0.001  LowerLimit=0+0.002
  Scope : Scope  NumInputPorts=2
  Sine : Lookup_n-D  NumberOfTableDimensions=1  LookupTableObject=''  BreakpointsForDimension1=[0:2*pi/4095:2*pi]  BreakpointsForDimension1FirstPoint=10  BreakpointsForDimension2FirstPoint=10  BreakpointsForDimension1Spacing=12  BreakpointsForDimension2Spacing=12  IndexSearchMethod=Evenly spaced points  Table=Sine_table  InterpMethod=Flat  DiagnosticForOutOfRangeInput=Error  InternalRulePriority=Speed  RndMeth=Simplest  InputSameDT=on
  Sin : Outport  VectorParamsAs1DForOutWhenUnconnected=off
  Cos : Outport  Port=2  VectorParamsAs1DForOutWhenUnconnected=off
  wires:
  P/1 -> Saturation/1  "position"
  Sine/1 -> Scope/1, Sin/1
  Cosine/1 -> Scope/2, Cos/1
  Saturation/1 -> Cosine/1, Sine/1

== system PMSM_FOC_Tractio/Motor_Control/Motor_Control_Funtion/FOC_Control_100us/FOC/HF_Observer/HFI_Function/IPD/Theta_cacl/If Action Subsystem1 ==
  In1 : Inport
  Action Port : ActionPort  ActionPortLabel=elseif((u3>u1)&(u1>u2))
  Fcn : Fcn  Expr=(u(3)-u(1))/(u(3)-u(2))*30+30
  Out1 : Outport
  wires:
  In1/1 -> Fcn/1
  Fcn/1 -> Out1/1

== system PMSM_FOC_Tractio/Motor_Control/Motor_Control_Funtion/FOC_Control_100us/FOC/HF_Observer/HFI_Function/IPD/Theta_cacl/If Action Subsystem2 ==
  In1 : Inport
  Action Port : ActionPort  ActionPortLabel=if((u1>u3)&(u3>u2))
  Fcn : Fcn  Expr=(u(3)-u(2))/(u(1)-u(2))*30
  Out1 : Outport
  wires:
  In1/1 -> Fcn/1
  Fcn/1 -> Out1/1

== system PMSM_FOC_Tractio/Motor_Control/Motor_Control_Funtion/FOC_Control_100us/FOC/HF_Observer/HFI_Function/IPD/Theta_cacl/If Action Subsystem3 ==
  In1 : Inport
  Action Port : ActionPort  ActionPortLabel=elseif((u3>u2)&(u2>u1))
  Fcn : Fcn  Expr=(u(2)-u(1))/(u(3)-u(1))*30+60
  Out1 : Outport
  wires:
  In1/1 -> Fcn/1
  Fcn/1 -> Out1/1

== system PMSM_FOC_Tractio/Motor_Control/Motor_Control_Funtion/FOC_Control_100us/FOC/HF_Observer/HFI_Function/IPD/Theta_cacl/If Action Subsystem4 ==
  In1 : Inport
  Action Port : ActionPort  ActionPortLabel=elseif((u2>u3)&(u3>u1))
  Fcn : Fcn  Expr=(u(2)-u(3))/(u(2)-u(1))*30+90
  Out1 : Outport
  wires:
  In1/1 -> Fcn/1
  Fcn/1 -> Out1/1

== system PMSM_FOC_Tractio/Motor_Control/Motor_Control_Funtion/FOC_Control_100us/FOC/HF_Observer/HFI_Function/IPD/Theta_cacl/If Action Subsystem5 ==
  In1 : Inport
  Action Port : ActionPort  ActionPortLabel=elseif((u2>u1)&(u1>u3))
  Fcn : Fcn  Expr=(u(1)-u(3))/(u(2)-u(3))*30+120
  Out1 : Outport
  wires:
  In1/1 -> Fcn/1
  Fcn/1 -> Out1/1

== system PMSM_FOC_Tractio/Motor_Control/Motor_Control_Funtion/FOC_Control_100us/FOC/HF_Observer/HFI_Function/IPD/Theta_cacl/If Action Subsystem6 ==
  In1 : Inport
  Action Port : ActionPort  ActionPortLabel=elseif((u1>u2)&(u2>u3))
  Fcn : Fcn  Expr=(u(1)-u(2))/(u(1)-u(3))*30+150
  Out1 : Outport
  wires:
  In1/1 -> Fcn/1
  Fcn/1 -> Out1/1

== system PMSM_FOC_Tractio/Motor_Control/Motor_Control_Funtion/FOC_Control_100us/FOC/HF_Observer/HFI_Function/NS/Ud_inject_1/Sine_Cosine ==
  note: Sine Cosine Coefficients
  P : Inport
  Cosine : Lookup_n-D  NumberOfTableDimensions=1  LookupTableObject=''  BreakpointsForDimension1=[0:2*pi/4095:2*pi]  BreakpointsForDimension1FirstPoint=10  BreakpointsForDimension2FirstPoint=10  BreakpointsForDimension1Spacing=12  BreakpointsForDimension2Spacing=12  IndexSearchMethod=Evenly spaced points  Table=Cosine_table  InterpMethod=Flat  DiagnosticForOutOfRangeInput=Error  InternalRulePriority=Speed  RndMeth=Simplest  InputSameDT=on
  Scope : Scope  NumInputPorts=2
  Sine : Lookup_n-D  NumberOfTableDimensions=1  LookupTableObject=''  BreakpointsForDimension1=[0:2*pi/4095:2*pi]  BreakpointsForDimension1FirstPoint=10  BreakpointsForDimension2FirstPoint=10  BreakpointsForDimension1Spacing=12  BreakpointsForDimension2Spacing=12  IndexSearchMethod=Evenly spaced points  Table=Sine_table  InterpMethod=Flat  DiagnosticForOutOfRangeInput=Error  InternalRulePriority=Speed  RndMeth=Simplest  InputSameDT=on
  Sin : Outport  VectorParamsAs1DForOutWhenUnconnected=off
  Cos : Outport  Port=2  VectorParamsAs1DForOutWhenUnconnected=off
  wires:
  P/1 -> Cosine/1, Sine/1  "position"
  Sine/1 -> Scope/1, Sin/1
  Cosine/1 -> Scope/2, Cos/1

== system PMSM_FOC_Tractio/Motor_Control/Motor_Control_Funtion/FOC_Control_100us/FOC/HF_Observer/HFI_Function/NS/Ud_inject_2/Sine_Cosine ==
  note: Sine Cosine Coefficients
  P : Inport
  Cosine : Lookup_n-D  NumberOfTableDimensions=1  LookupTableObject=''  BreakpointsForDimension1=[0:2*pi/4095:2*pi]  BreakpointsForDimension1FirstPoint=10  BreakpointsForDimension2FirstPoint=10  BreakpointsForDimension1Spacing=12  BreakpointsForDimension2Spacing=12  IndexSearchMethod=Evenly spaced points  Table=Cosine_table  InterpMethod=Flat  DiagnosticForOutOfRangeInput=Error  InternalRulePriority=Speed  RndMeth=Simplest  InputSameDT=on
  Scope : Scope  NumInputPorts=2
  Sine : Lookup_n-D  NumberOfTableDimensions=1  LookupTableObject=''  BreakpointsForDimension1=[0:2*pi/4095:2*pi]  BreakpointsForDimension1FirstPoint=10  BreakpointsForDimension2FirstPoint=10  BreakpointsForDimension1Spacing=12  BreakpointsForDimension2Spacing=12  IndexSearchMethod=Evenly spaced points  Table=Sine_table  InterpMethod=Flat  DiagnosticForOutOfRangeInput=Error  InternalRulePriority=Speed  RndMeth=Simplest  InputSameDT=on
  Sin : Outport  VectorParamsAs1DForOutWhenUnconnected=off
  Cos : Outport  Port=2  VectorParamsAs1DForOutWhenUnconnected=off
  wires:
  P/1 -> Cosine/1, Sine/1  "position"
  Sine/1 -> Scope/1, Sin/1
  Cosine/1 -> Scope/2, Cos/1

== system PMSM_FOC_Tractio/Motor_Control/Motor_Control_Funtion/FOC_Control_100us/FOC/HF_Observer/HFI_Function/NS/Ud_inject_3/Sine_Cosine ==
  note: Sine Cosine Coefficients
  P : Inport
  Cosine : Lookup_n-D  NumberOfTableDimensions=1  LookupTableObject=''  BreakpointsForDimension1=[0:2*pi/4095:2*pi]  BreakpointsForDimension1FirstPoint=10  BreakpointsForDimension2FirstPoint=10  BreakpointsForDimension1Spacing=12  BreakpointsForDimension2Spacing=12  IndexSearchMethod=Evenly spaced points  Table=Cosine_table  InterpMethod=Flat  DiagnosticForOutOfRangeInput=Error  InternalRulePriority=Speed  RndMeth=Simplest  InputSameDT=on
  Scope : Scope  NumInputPorts=2
  Sine : Lookup_n-D  NumberOfTableDimensions=1  LookupTableObject=''  BreakpointsForDimension1=[0:2*pi/4095:2*pi]  BreakpointsForDimension1FirstPoint=10  BreakpointsForDimension2FirstPoint=10  BreakpointsForDimension1Spacing=12  BreakpointsForDimension2Spacing=12  IndexSearchMethod=Evenly spaced points  Table=Sine_table  InterpMethod=Flat  DiagnosticForOutOfRangeInput=Error  InternalRulePriority=Speed  RndMeth=Simplest  InputSameDT=on
  Sin : Outport  VectorParamsAs1DForOutWhenUnconnected=off
  Cos : Outport  Port=2  VectorParamsAs1DForOutWhenUnconnected=off
  wires:
  P/1 -> Cosine/1, Sine/1  "position"
  Sine/1 -> Scope/1, Sin/1
  Cosine/1 -> Scope/2, Cos/1

== system PMSM_FOC_Tractio/Motor_Control/Motor_Control_Funtion/FOC_Control_100us/FOC/HF_Observer/HFI_Function/NS/Ud_inject_4/Sine_Cosine ==
  note: Sine Cosine Coefficients
  P : Inport
  Cosine : Lookup_n-D  NumberOfTableDimensions=1  LookupTableObject=''  BreakpointsForDimension1=[0:2*pi/4095:2*pi]  BreakpointsForDimension1FirstPoint=10  BreakpointsForDimension2FirstPoint=10  BreakpointsForDimension1Spacing=12  BreakpointsForDimension2Spacing=12  IndexSearchMethod=Evenly spaced points  Table=Cosine_table  InterpMethod=Flat  DiagnosticForOutOfRangeInput=Error  InternalRulePriority=Speed  RndMeth=Simplest  InputSameDT=on
  Scope : Scope  NumInputPorts=2
  Sine : Lookup_n-D  NumberOfTableDimensions=1  LookupTableObject=''  BreakpointsForDimension1=[0:2*pi/4095:2*pi]  BreakpointsForDimension1FirstPoint=10  BreakpointsForDimension2FirstPoint=10  BreakpointsForDimension1Spacing=12  BreakpointsForDimension2Spacing=12  IndexSearchMethod=Evenly spaced points  Table=Sine_table  InterpMethod=Flat  DiagnosticForOutOfRangeInput=Error  InternalRulePriority=Speed  RndMeth=Simplest  InputSameDT=on
  Sin : Outport  VectorParamsAs1DForOutWhenUnconnected=off
  Cos : Outport  Port=2  VectorParamsAs1DForOutWhenUnconnected=off
  wires:
  P/1 -> Cosine/1, Sine/1  "position"
  Sine/1 -> Scope/1, Sin/1
  Cosine/1 -> Scope/2, Cos/1

== system PMSM_FOC_Tractio/Motor_Control/Motor_Control_Funtion/FOC_Control_100us/FOC/HF_Observer/HFI_Function/NS/Ud_inject_4/Theta_limit ==
  Angle_input : Inport
  Angle_offset : Constant  Value=pi  OutDataTypeStr=single
  If Action Subsystem1 : Subsystem  TreatAsAtomicUnit=on
  If Action Subsystem2 : Subsystem  TreatAsAtomicUnit=on
  If1 : If  IfExpression=u1 > 6.283185307
  Merge1 : Merge
  Subtract1 : Sum
  Angle_output : Outport
  wires:
  Angle_input/1 -> Subtract1/1
  Merge1/1 -> Angle_output/1
  Angle_offset/1 -> Subtract1/2
  If1/1 -> If Action Subsystem2/Action
  If1/2 -> If Action Subsystem1/Action
  If Action Subsystem2/1(Out1) -> Merge1/1
  Subtract1/1 -> If Action Subsystem1/1(In1), If Action Subsystem2/1(In1), If1/1
  If Action Subsystem1/1(Out1) -> Merge1/2

== system PMSM_FOC_Tractio/Motor_Control/Motor_Control_Funtion/FOC_Control_100us/FOC/HF_Observer/HFI_Function/NS/Ud_inject_5/Sine_Cosine ==
  note: Sine Cosine Coefficients
  P : Inport
  Cosine : Lookup_n-D  NumberOfTableDimensions=1  LookupTableObject=''  BreakpointsForDimension1=[0:2*pi/4095:2*pi]  BreakpointsForDimension1FirstPoint=10  BreakpointsForDimension2FirstPoint=10  BreakpointsForDimension1Spacing=12  BreakpointsForDimension2Spacing=12  IndexSearchMethod=Evenly spaced points  Table=Cosine_table  InterpMethod=Flat  DiagnosticForOutOfRangeInput=Error  InternalRulePriority=Speed  RndMeth=Simplest  InputSameDT=on
  Scope : Scope  NumInputPorts=2
  Sine : Lookup_n-D  NumberOfTableDimensions=1  LookupTableObject=''  BreakpointsForDimension1=[0:2*pi/4095:2*pi]  BreakpointsForDimension1FirstPoint=10  BreakpointsForDimension2FirstPoint=10  BreakpointsForDimension1Spacing=12  BreakpointsForDimension2Spacing=12  IndexSearchMethod=Evenly spaced points  Table=Sine_table  InterpMethod=Flat  DiagnosticForOutOfRangeInput=Error  InternalRulePriority=Speed  RndMeth=Simplest  InputSameDT=on
  Sin : Outport  VectorParamsAs1DForOutWhenUnconnected=off
  Cos : Outport  Port=2  VectorParamsAs1DForOutWhenUnconnected=off
  wires:
  P/1 -> Cosine/1, Sine/1  "position"
  Sine/1 -> Scope/1, Sin/1
  Cosine/1 -> Scope/2, Cos/1

== system PMSM_FOC_Tractio/Motor_Control/Motor_Control_Funtion/FOC_Control_100us/FOC/HF_Observer/HFI_Function/NS/Ud_inject_5/Subsystem ==
  In1 : Inport
  Action Port : ActionPort  ActionPortLabel=if(u1>=u2)
  Out1 : Outport
  wires:
  In1/1 -> Out1/1

== system PMSM_FOC_Tractio/Motor_Control/Motor_Control_Funtion/FOC_Control_100us/FOC/HF_Observer/HFI_Function/NS/Ud_inject_5/Subsystem1 ==
  In1 : Inport
  Action Port : ActionPort  ActionPortLabel=elseif(u1<u2)
  Theta_limit : Subsystem
      settings: RTWSystemCode=Nonreusable function  RTWFcnNameOpts=Use subsystem name
  Out1 : Outport
  wires:
  In1/1 -> Theta_limit/1(Angle_input)
  Theta_limit/1(Angle_output) -> Out1/1

== system PMSM_FOC_Tractio/Motor_Control/Motor_Control_Funtion/FOC_Control_100us/FOC/HF_Observer/HFI_Function/HFI/IPD_Angle/Angle_calibration/If Action Subsystem1 ==
  In1 : Inport
  Action Port : ActionPort  ActionPortLabel=else
  Out1 : Outport
  wires:
  In1/1 -> Out1/1

== system PMSM_FOC_Tractio/Motor_Control/Motor_Control_Funtion/FOC_Control_100us/FOC/HF_Observer/HFI_Function/HFI/IPD_Angle/Angle_calibration/If Action Subsystem2 ==
  In1 : Inport
  Action Port : ActionPort  ActionPortLabel=if(u1 > 6.283185307)
  2pi : Constant  Value=2*pi  OutDataTypeStr=single
  Subtract1 : Sum  Inputs=+-  OutDataTypeStr=single
  Out1 : Outport
  wires:
  In1/1 -> Subtract1/1
  Subtract1/1 -> Out1/1
  2pi/1 -> Subtract1/2

== system PMSM_FOC_Tractio/Motor_Control/Motor_Control_Funtion/FOC_Control_100us/FOC/HF_Observer/HFI_Function/HFI/IPD_Angle/Angle_calibration/If Action Subsystem3 ==
  In1 : Inport
  Action Port : ActionPort  ActionPortLabel=elseif(u1<0)
  Angle_offset : Constant  Value=2*pi  OutDataTypeStr=single
  Subtract1 : Sum
  Out1 : Outport
  wires:
  In1/1 -> Subtract1/1
  Subtract1/1 -> Out1/1
  Angle_offset/1 -> Subtract1/2

== system PMSM_FOC_Tractio/Motor_Control/Motor_Control_Funtion/FOC_Control_100us/FOC/HF_Observer/HFI_Function/HFI/IPD_Angle1/Angle_calibration/If Action Subsystem1 ==
  In1 : Inport
  Action Port : ActionPort  ActionPortLabel=else
  Out1 : Outport
  wires:
  In1/1 -> Out1/1

== system PMSM_FOC_Tractio/Motor_Control/Motor_Control_Funtion/FOC_Control_100us/FOC/HF_Observer/HFI_Function/HFI/IPD_Angle1/Angle_calibration/If Action Subsystem2 ==
  In1 : Inport
  Action Port : ActionPort  ActionPortLabel=if(u1 > 6.283185307)
  2pi : Constant  Value=2*pi  OutDataTypeStr=single
  Subtract1 : Sum  Inputs=+-  OutDataTypeStr=single
  Out1 : Outport
  wires:
  In1/1 -> Subtract1/1
  Subtract1/1 -> Out1/1
  2pi/1 -> Subtract1/2

== system PMSM_FOC_Tractio/Motor_Control/Motor_Control_Funtion/FOC_Control_100us/FOC/HF_Observer/HFI_Function/HFI/IPD_Angle1/Angle_calibration/If Action Subsystem3 ==
  In1 : Inport
  Action Port : ActionPort  ActionPortLabel=elseif(u1<0)
  Angle_offset : Constant  Value=2*pi  OutDataTypeStr=single
  Subtract1 : Sum
  Out1 : Outport
  wires:
  In1/1 -> Subtract1/1
  Subtract1/1 -> Out1/1
  Angle_offset/1 -> Subtract1/2

== system PMSM_FOC_Tractio/Motor_Control/Motor_Control_Funtion/FOC_Control_100us/FOC/HF_Observer/HFI_Function/NS/Ud_inject_4/Theta_limit/If Action Subsystem1 ==
  In1 : Inport
  Action Port : ActionPort  ActionPortLabel=else
  Out1 : Outport
  wires:
  In1/1 -> Out1/1

== system PMSM_FOC_Tractio/Motor_Control/Motor_Control_Funtion/FOC_Control_100us/FOC/HF_Observer/HFI_Function/NS/Ud_inject_4/Theta_limit/If Action Subsystem2 ==
  In1 : Inport
  Action Port : ActionPort  ActionPortLabel=if(u1 > 6.283185307)
  2pi : Constant  Value=2*pi  OutDataTypeStr=single
  Subtract1 : Sum  Inputs=+-
  Out1 : Outport
  wires:
  In1/1 -> Subtract1/1
  Subtract1/1 -> Out1/1
  2pi/1 -> Subtract1/2

== system PMSM_FOC_Tractio/Motor_Control/Motor_Control_Funtion/FOC_Control_100us/FOC/HF_Observer/HFI_Function/NS/Ud_inject_5/Subsystem1/Theta_limit ==
  Angle_input : Inport
  Angle_offset : Constant  Value=pi  OutDataTypeStr=single
  If Action Subsystem1 : Subsystem  TreatAsAtomicUnit=on
  If Action Subsystem2 : Subsystem  TreatAsAtomicUnit=on
  If1 : If  IfExpression=u1 > 6.283185307
  Merge1 : Merge
  Subtract1 : Sum
  Angle_output : Outport
  wires:
  Angle_input/1 -> Subtract1/1
  Merge1/1 -> Angle_output/1
  Angle_offset/1 -> Subtract1/2
  If1/1 -> If Action Subsystem2/Action
  If1/2 -> If Action Subsystem1/Action
  If Action Subsystem2/1(Out1) -> Merge1/1
  Subtract1/1 -> If Action Subsystem1/1(In1), If Action Subsystem2/1(In1), If1/1
  If Action Subsystem1/1(Out1) -> Merge1/2

== system PMSM_FOC_Tractio/Motor_Control/Motor_Control_Funtion/FOC_Control_100us/FOC/HF_Observer/HFI_Function/NS/Ud_inject_5/Subsystem1/Theta_limit/If Action Subsystem1 ==
  In1 : Inport
  Action Port : ActionPort  ActionPortLabel=else
  Out1 : Outport
  wires:
  In1/1 -> Out1/1

== system PMSM_FOC_Tractio/Motor_Control/Motor_Control_Funtion/FOC_Control_100us/FOC/HF_Observer/HFI_Function/NS/Ud_inject_5/Subsystem1/Theta_limit/If Action Subsystem2 ==
  In1 : Inport
  Action Port : ActionPort  ActionPortLabel=if(u1 > 6.283185307)
  2pi : Constant  Value=2*pi  OutDataTypeStr=single
  Subtract1 : Sum  Inputs=+-
  Out1 : Outport
  wires:
  In1/1 -> Subtract1/1
  Subtract1/1 -> Out1/1
  2pi/1 -> Subtract1/2

== stateflow chart PMSM_FOC_Tractio/Motor_Control/Motor_Control_Funtion/Angle_Speed_100us/SpeedAndAngle/Chart ==
  state BLDC_State
    en,du:
    BLDC_LOCK_Flag=1;
    BLDC_State=1;
  state BLDC_RUN
    en,du:
    BLDC_State=2;
  state BLDC_Switch
    BLDC_State=3;
  (default) -> BLDC_State
  BLDC_State -> BLDC_RUN : [after(0.01,sec) &&BLDC_State==1 ]
  BLDC_RUN -> BLDC_Switch : [after(0.2,sec) &&BLDC_State==2]
  data: BLDC_LOCK_Flag local; BLDC_RUN_Flag local; BLDC_State output uint8

== stateflow chart PMSM_FOC_Tractio/Motor_Control/Motor_Control_Funtion/Angle_Speed_100us/State_machine ==
  state Motor_Stop
    entry: Motor_state = 0;
  state Motor_Start
    en: Motor_state = 1;
    OPL_flag=1;
  state Motor_OPL
    en: Motor_state=2;
    CL_flag=1;
  state Motor_CL
    en:Motor_state=3;
  state Motor_CL1
    en:Motor_state=4;
  (default) -> Motor_Start
  Motor_Start -> Motor_OPL [order 2] : [Sensorless_flag==1]
  Motor_Stop -> Motor_Start : [Sensorless_flag==1]
  Motor_Start -> Motor_Stop [order 1] : [Sensorless_flag==0]
  Motor_OPL -> Motor_CL [order 1] : [after(OPL_Param.Acc_Times,sec) & Sensorless_flag==1 & CL_flag==1 & Speed_Measured>(OPL_Param.Target_RPM-100)]
  Motor_OPL -> Motor_Stop [order 2] : [Sensorless_flag==0]
  Motor_CL1 -> Motor_Stop : [Sensorless_flag==0]
  Motor_CL -> Motor_Stop [order 1] : [Sensorless_flag==0]
  Motor_CL -> Motor_CL1 [order 2] : [after(OPL_Param.Revup_Times,sec) & Sensorless_flag==1]
  data: Sensorless_flag input; Motor_state output uint8; OPL_flag local; Speed_Measured input; CL_flag local; OPL_Param parameter

== stateflow chart PMSM_FOC_Tractio/Motor_Control/Motor_Control_Funtion/FOC_Control_100us/FOC/HF_Observer/HFI_Function/HFI/StartRUN_State_machine ==
  note: [RUN_flag==1]
  state NS_2_RUN
    en: RUN_state = 1;
    NS_RUN_flag=1;
  state Start_RUN
    en: RUN_state=2;
    Switch_flag=1;
  state RUN
    en: RUN_state=3;
    Start_RUN_flag=1;
  (default) -> NS_2_RUN
  NS_2_RUN -> Start_RUN : [after(HFI.NS2RUN_Time,sec) &NS_RUN_flag==1]
  Start_RUN -> RUN : [after(HFI.Switch_Time,sec) &Switch_flag==1]
  data: RUN_state output uint8; NS_RUN_flag local; Start_RUN_flag local; RUN_flag input; HFI parameter; Switch_flag local

== stateflow chart PMSM_FOC_Tractio/Motor_Control/Motor_Control_Funtion/FOC_Control_100us/FOC/HF_Observer/HFI_Function/HFI_State_machine ==
  note: [HFI_flag==1]
  state HFI_NS
    en: HFI_state=2;
    NS_flag=1;
  state HFI_IPD
    en: HFI_state = 1;
    IPD_flag=1;
  state HFI_RUN
    en:HFI_state=3;
    HFI_RUN_flag=1;
  (default) -> HFI_IPD
  HFI_IPD -> HFI_NS : [after(HFI.IPD_Time,sec) &HFI_flag==1 & IPD_flag==1]
  HFI_NS -> HFI_RUN : [after(HFI.NS_Time,sec) & NS_flag==1]
  data: HFI_flag input; HFI_state output uint8; IPD_flag local; NS_flag local; HFI_RUN_flag local; NS_RUN_flag local; HFI parameter
